simulink model "lab_4_task_1_simulink"  (R2025b)
settings: Solver=ode5  StartTime=0.0  StopTime=10.0  FixedStep=0.1  RelTol=1e-3
values from neighbouring files (symbols this model uses):
  A0 = eye(3)    [lab_4_task_1.m]    (also in lab_5_task_1.m; lab_5_task_2.m)
  I = diag([ix iy iz])    [lab_4_task_1.m]    (also in lab_5_task_1.m; lab_5_task_2.m; lab_6_task_1.m = diag([ ix iy iz ]); lab_6_task_2.m = diag([ ix iy iz ]))
  ix = 0.070    (= 0.07)    [lab_3_task_1.m]    (also in lab_3_task_2.m = 0.0504; lab_3_task_3.m = 0.025; lab_3_task_4.m; lab_4_task_1.m)
  iy = 0.055    [lab_3_task_1.m]    (also in lab_3_task_2.m = 0.0504; lab_3_task_3.m; lab_3_task_4.m = 0.0109; lab_4_task_1.m)
  iz = 0.025    [lab_3_task_1.m]    (also in lab_3_task_2.m = 0.0109; lab_3_task_3.m = 0.07; lab_3_task_4.m = 0.0504; lab_4_task_1.m)
  w0 = [0.01 0.01 0.01]    [lab_3_task_3.m]    (also in lab_5_task_1.m = [wx0 wy0 wz0]; lab_5_task_2.m = [wx0 wy0 wz0]; lab_6_task_1.m = [wx0 wy0 wz0]; lab_6_task_2.m = [wx0 wy0 wz0])
  wx0 = 0.45    [lab_3_task_1.m]    (also in lab_3_task_2.m = 0.1; lab_3_task_3.m = w0(1); lab_3_task_4.m = 1e-06; lab_4_task_1.m)
  wy0 = 0.52    [lab_3_task_1.m]    (also in lab_3_task_2.m = 0.1; lab_3_task_3.m = w0(2); lab_3_task_4.m = 1e-06; lab_4_task_1.m)
  wz0 = 0.55    [lab_3_task_1.m]    (also in lab_3_task_2.m = 0.1; lab_3_task_3.m = w0(3); lab_3_task_4.m = 0.02; lab_4_task_1.m)
libraries: matrix_library x1
settings Model: Creator=nicol  LastModifiedBy=nicol

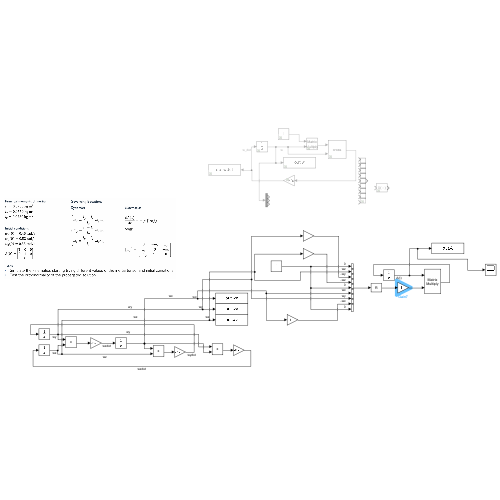
[thumbnail: Simulink's stored preview of the top-level diagram]
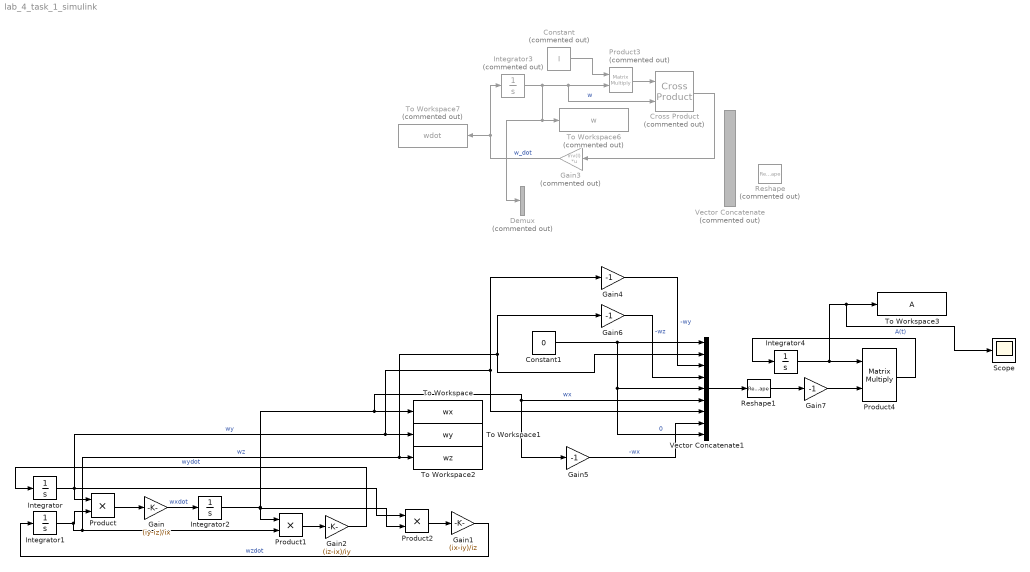
== system lab_4_task_1_simulink ==
  Constant : Constant  Commented=on  Value=I
  Constant1 : Constant  Value=0
  Cross Product : matrix_library/Cross Product  Commented=on
  Demux : Demux  Commented=on  Outputs=3
  Gain : Gain  Gain=(iy-iz)/ix
  Gain1 : Gain  Gain=(ix-iy)/iz
  Gain2 : Gain  Gain=(iz-ix)/iy
  Gain3 : Gain  Commented=on  Gain=inv(I)  Multiplication=Matrix(K*u)
  Gain{4..7} (4 alike) : Gain  Gain=-1
  Integrator : Integrator  InitialCondition=wy0
  Integrator1 : Integrator  InitialCondition=wz0
  Integrator2 : Integrator  InitialCondition=wx0
  Integrator3 : Integrator  Commented=on  InitialCondition=w0
  Integrator4 : Integrator  InitialCondition=A0
  Product : Product
  Product1 : Product
  Product2 : Product
  Product3 : Product  Commented=on  Multiplication=Matrix(*)
  Product4 : Product  Multiplication=Matrix(*)
  Reshape : Reshape  Commented=on
  Reshape1 : Reshape  OutputDimensionality=Customize  OutputDimensions=[3,3]
  Scope : Scope
      settings: ActiveDisplayYMinimum=-1.2451714263002922  ActiveDisplayYMaximum=1.2494634918111436
  To Workspace : ToWorkspace  VariableName=wx  SaveFormat=Timeseries  SampleTime=-1
  To Workspace1 : ToWorkspace  VariableName=wy  SaveFormat=Timeseries  SampleTime=-1
  To Workspace2 : ToWorkspace  VariableName=wz  SaveFormat=Timeseries  SampleTime=-1
  To Workspace3 : ToWorkspace  VariableName=A  SaveFormat=Timeseries  SampleTime=-1
  To Workspace6 : ToWorkspace  Commented=on  VariableName=w  SaveFormat=Timeseries  SampleTime=-1
  To Workspace7 : ToWorkspace  Commented=on  VariableName=wdot  SaveFormat=Timeseries  SampleTime=-1
  Vector Concatenate : Concatenate  Commented=on  NumInputs=9
  Vector Concatenate1 : Concatenate  NumInputs=9
  wires:
  Product3/1 -> Cross Product/1
  Integrator3/1 -> To Workspace6/1, Demux/1, Cross Product/2, Product3/2  "w"
  Constant/1 -> Product3/1
  Cross Product/1 -> Gain3/1
  Gain3/1 -> Integrator3/1, To Workspace7/1  "w_dot"
  Gain2/1 -> Integrator/1  "wydot"
  Integrator1/1 -> Gain6/1, Vector Concatenate1/2, To Workspace2/1, Product1/2, Product/2  "wz"
  Gain/1 -> Integrator2/1  "wxdot"
  Product1/1 -> Gain2/1
  Integrator2/1 -> Product2/2, Product1/1, Gain5/1, Vector Concatenate1/6, To Workspace/1  "wx"
  Gain1/1 -> Integrator1/1  "wzdot"
  Product/1 -> Gain/1
  Integrator/1 -> Gain4/1, Vector Concatenate1/7, To Workspace1/1, Product2/1, Product/1  "wy"
  Product2/1 -> Gain1/1
  Constant1/1 -> Vector Concatenate1/9, Vector Concatenate1/5, Vector Concatenate1/1  "0"
  Gain5/1 -> Vector Concatenate1/8  "-wx"
  Gain4/1 -> Vector Concatenate1/3  "-wy"
  Gain6/1 -> Vector Concatenate1/4  "-wz"
  Vector Concatenate1/1 -> Reshape1/1
  Product4/1 -> Integrator4/1
  Integrator4/1 -> Scope/1, To Workspace3/1, Product4/1  "A(t)"
  Reshape1/1 -> Gain7/1
  Gain7/1 -> Product4/2
